simulink model "Quadcopter_close_loop"  (R2021a)
settings: Solver=ode4  StartTime=0.0  StopTime=87  FixedStep=0.001  RelTol=1e-6
values from neighbouring files (symbols this model uses):
  mean_wind = [2.72 , 1.75, -0.006]    [main_run.m]    (also in main_run_5_1.m; param_est.m = [2.72 , 1.75, .006])
  q = X(7:10)    [EKF_without_wind.m]
  r = linspace(floor(nr*0.01)/nr,1,nr)    [main_run.m]    (also in main_run_5_1.m)
  w1 = w(1)    [EKF_without_wind.m]
  x0 = [0,0,0,1,0,0,0,-P.mean_wind,0,0,0]    [main_run.m]    (also in main_run_5_1.m)
  xref = [1,1,-8,1,0,0,0,-P.mean_wind]    [main_run.m]    (also in main_run_5_1.m)
undefined symbols (not defined in the file or in its folder): HDBK, MIL, Moderate, P, u1, v1
libraries: simulink x1, aerolibwind2 x1
(part 2 of 5)

== matlab function Quadcopter_close_loop/Estimator/Estimator/IEKF_quadcopter ==
  data: sensor input; t input; y output; P parameter
function y = IEKF_quadcopter(sensor,t,P)
%% parameters 
ts = 0.01;
m = P.m;
g = P.g;
rho = P.rho;
D = P.D;
A_gr = [0;0;g];
B_i = P.B_i;

param = cell(1,6);
param{1} = A_gr;
param{2} = m;
param{3} = rho;
param{4} = D;
param{5} = ts;
param{6} = B_i;

Q_est = P.Q_est;
R_est = P.R_est;
X0_hat = P.X0_hat;
IEKF_P0 = P.IEKF_P0;
%% IEKF
persistent k P_cov X

if t >=0
    if isempty(k)
        k = 1;
        X = zeros(13,1);
        [X,P_cov] = IEKF(X0_hat,IEKF_P0,Q_est,R_est,param,sensor,k);
    end
    k = k+1;
    [X,P_cov] = IEKF(X,P_cov,Q_est,R_est,param,sensor,k);
else
    X = zeros(13,1);
end

quat = X(7:10);  
eul = quat2eul(quat')';
eul([1 3]) = eul([3 1]);
X_est = [X(1:6);eul;X(11:13)];
% Asma: Dynamics states: pos, quaternion, velocity, wind? Rearranged the dynamics so that it goes into contoller correctly 

% X_est=[X(1:3); X(7:10); X(4:6); X(11:13)];

y=X_est;
end

function [X_k1,P_k1] = IEKF(X,P,Q,R,param,sensor,iter)
% Performs one loop of the SP-EKF.
% Pre-Observer is of the form:
%   Xhat_dot = f(Xhat) + Fr*L*E*(Y - Yhat)

% Inputs:

%   X = State mean, m_k|k-1 (nx1)
%   P = State covariance, P_k|k-1(nxn)
%   f = State dynamics, xdot = f(x,param)
%   df = 
%   dh =
%   Q = Process Noise Covariance Matrix(nxn)
%   R = Measurement Noise Covariance Matrix (mxm)
%   param = Any parameters for f
%   iter = denotes the the first loop,1=yes,0=no

% Outputs:

%   X_k1 = state at next time step
%   P_k1 = state covariance at next time step

%parameter
A_gr = param{1};
m = param{2};
rho = param{3};
D = param{4};
ts = param{5};
B_i = param{6};
%sensor
% Y=[sensor{1};sensor{2};sensor{3}]; %gps+accel+B_b
% w = sensor{4};
% f_c = sensor{5};
gps = sensor(1:3);
accel = sensor(4:6);
w = sensor(7:9);
B_b = sensor(10:12);
f_c = sensor(13);

Y=[gps;accel;B_b];
U={w;f_c}; %w+f_c
%states(13*1)
x_hat=X(1:3);
vr_hat=X(4:6);
q_hat=X(7:10);
d_hat=X(11:13);

vr_hat1=vr_hat(1);vr_hat2=vr_hat(2);vr_hat3=vr_hat(3);
q_hat0=q_hat(1);q_hat1=q_hat(2);q_hat2=q_hat(3);q_hat3=q_hat(4);
%invariants
I_vr = quat_v(q_hat,vr_hat,0);
I_w = quat_v(q_hat,w,0);
b3=[0;0;1];
I_f_c = quat_v(q_hat,f_c*b3,0);
%state matrix needed for implementing the IEKF(linearized A matrix)
if norm(I_vr)==0
    mid_element=zeros(3,3);
else
%         I_D= quat_m(q_hat,D,0);
      I_D =D;
      I_D= quat_D(q_hat,D);
    mid_element =-0.5*(1/m)*rho*I_D*[norm(I_vr)+(I_vr(1)*abs(I_vr(1))*sign(I_vr(1)))/norm(I_vr)... 
                                              (I_vr(1)*abs(I_vr(2))*sign(I_vr(2)))/norm(I_vr)...
                                              (I_vr(1)*abs(I_vr(3))*sign(I_vr(3)))/norm(I_vr); ...
                                              (I_vr(2)*abs(I_vr(1))*sign(I_vr(1)))/norm(I_vr) ...
                                   norm(I_vr)+(I_vr(2)*abs(I_vr(2))*sign(I_vr(2)))/norm(I_vr) ...
                                              (I_vr(2)*abs(I_vr(3))*sign(I_vr(3)))/norm(I_vr);...
                                              (I_vr(3)*abs(I_vr(1))*sign(I_vr(1)))/norm(I_vr) ...
                                              (I_vr(3)*abs(I_vr(2))*sign(I_vr(2)))/norm(I_vr) ...
                                   norm(I_vr)+(I_vr(3)*abs(I_vr(3))*sign(I_vr(3)))/norm(I_vr);]; 
end

%dim=12x12
A_lin =@(I_vr,A_gr)[zeros(3,3)      eye(3)  -2*hat(I_vr)     eye(3);...
                    zeros(3,3) mid_element   2*hat(A_gr) zeros(3,3);...
                    zeros(3,3)  zeros(3,3)    zeros(3,3) zeros(3,3);...
                    zeros(3,3)  zeros(3,3)    zeros(3,3) zeros(3,3);]; 

%Invariant frame (13x12)
Fr =@(q_hat)[    eye(3)      zeros(3,3)      zeros(3,3) zeros(3,3);
             zeros(3,3) quat_e(q_hat,0)      zeros(3,3) zeros(3,3);
             zeros(4,3)      zeros(4,3) quat_e(q_hat,2) zeros(4,3);
             zeros(3,3)      zeros(3,3)      zeros(3,3)    eye(3);]; 
    

%T = Invariant Output Matrix, (9x9)
T =@(q_hat) [    eye(3)          zeros(3,3)    zeros(3,3);
             zeros(3,3)    quat_e(q_hat,1)     zeros(3,3);
             zeros(3,3)        zeros(3,3)  quat_e(q_hat,1)]; 
         

Ln_22 = [vr_hat2*(2*q_hat0*q_hat2 + 2*q_hat1*q_hat3) + vr_hat3*(2*q_hat0*q_hat3 - 2*q_hat1*q_hat2),     - vr_hat3*(2*q_hat2^2 + 2*q_hat3^2 - 1) - vr_hat1*(2*q_hat0*q_hat2 + 2*q_hat1*q_hat3),       vr_hat2*(2*q_hat2^2 + 2*q_hat3^2 - 1) - vr_hat1*(2*q_hat0*q_hat3 - 2*q_hat1*q_hat2);
         vr_hat3*(2*q_hat1^2 + 2*q_hat3^2 - 1) - vr_hat2*(2*q_hat0*q_hat1 - 2*q_hat2*q_hat3), vr_hat1*(2*q_hat0*q_hat1 - 2*q_hat2*q_hat3) + vr_hat3*(2*q_hat0*q_hat3 + 2*q_hat1*q_hat2),     - vr_hat1*(2*q_hat1^2 + 2*q_hat3^2 - 1) - vr_hat2*(2*q_hat0*q_hat3 + 2*q_hat1*q_hat2);
         - vr_hat2*(2*q_hat1^2 + 2*q_hat2^2 - 1) - vr_hat3*(2*q_hat0*q_hat1 + 2*q_hat2*q_hat3),       vr_hat1*(2*q_hat1^2 + 2*q_hat2^2 - 1) - vr_hat3*(2*q_hat0*q_hat2 - 2*q_hat1*q_hat3), vr_hat1*(2*q_hat0*q_hat1 + 2*q_hat2*q_hat3) + vr_hat2*(2*q_hat0*q_hat2 - 2*q_hat1*q_hat3);];
Ln_23 = [ (2*q_hat0*q_hat2 + 2*q_hat1*q_hat3)/m;
         -(2*q_hat0*q_hat1 - 2*q_hat2*q_hat3)/m;
               -(2*q_hat1^2 + 2*q_hat2^2 - 1)/m;];
Ln_32 = [      q_hat2^2 + q_hat3^2 - 1/2,   q_hat0*q_hat3 - q_hat1*q_hat2, - q_hat0*q_hat2 - q_hat1*q_hat3;
         - q_hat0*q_hat3 - q_hat1*q_hat2,       q_hat1^2 + q_hat3^2 - 1/2,   q_hat0*q_hat1 - q_hat2*q_hat3;
          q_hat0*q_hat2 - q_hat1*q_hat3, - q_hat0*q_hat1 - q_hat2*q_hat3,       q_hat1^2 + q_hat2^2 - 1/2;];
% (12x10)
Ln =[   -eye(3)      zeros(3,3)    zeros(3,1) zeros(3,3);
     zeros(3,3)          Ln_22         Ln_23  zeros(3,3);
     zeros(3,3)          Ln_32     zeros(3,1) zeros(3,3);
     zeros(3,3)      zeros(3,3)    zeros(3,1)    -eye(3);]; 
 
 if iter ==1
    W=Fr(q_hat);
    W(7,:)=[];
    P = W'*P*W;
 end
%% time update 
    %continuous
    X_minus_k1 = X; %dim(X)=13x1
    P_minus_k1 = P; %dim(P)=12x12
    N=10;
    for i=1:N
    X_minus_k1 =X_minus_k1 + (ts/N).*f(X_minus_k1,U,param);
    
    %updated states and invariants
    q_hat=X_minus_k1(7:10);
    q_hat=q_hat/norm(q_hat);    
    X_minus_k1(7:10)=q_hat; %normalization
    vr_hat=X_minus_k1(4:6);
    I_vr=quat_v(q_hat,vr_hat,0);
    
    A=A_lin(I_vr,A_gr);
    P_minus_k1 = P_minus_k1 + (ts/N).*(A*P_minus_k1 + P_minus_k1*A' + Ln*Q*Ln');
    end
    X_k1 = X_minus_k1;
    P_k1 = P_minus_k1;
% measurement update 
    H= dh(X_minus_k1,U,param); %dim(H)=9x12
    R_rot = T(q_hat)*R*T(q_hat)';
    L = P_minus_k1*H'*inv(H*P_minus_k1*H' + R_rot); %dim(L)=12x9
%     L = P_minus_k1*H'*inv(H*P_minus_k1*H' + R); %dim(L)=12x9
%     X_k1 = X_minus_k1 + Fr(q_hat)*L_*T(q_hat)*(Y-H*X_minus_k1); %dim(X_k1)=13x1
    X_k1 = X_minus_k1 + Fr(q_hat)*L*T(q_hat)*(Y-h(X_minus_k1,U,param)); %dim(X_k1)=13x1
    
    q_hat=X_k1(7:10);
    q_hat=q_hat/norm(q_hat);    
    X_k1(7:10)=q_hat;
    
    P_k1 = (eye(12)-L*H)*P_minus_k1; %dim(P_k1) = 12x12
end
 
function [X_dot] = f(X,U,param)
%states
x=X(1:3);
vr=X(4:6);
q=X(7:10);
d=X(11:13);
%inputs
w=U{1};
f_c=U{2};
%parameters
A_gr = param{1};
m = param{2};
rho = param{3};
D = param{4};
ts = param{5};
B_i= param{6};
b_3=[0;0;1];
%% system dynamics
f_vr=-(1/2)*rho*D*norm(vr)*vr;
x_dot = quat_v(q,vr,0) + d;
vr_dot = cross(vr,w) + quat_v(q,A_gr,1) - (1/m)*f_c*b_3 + (1/m)*f_vr;
q_dot = (1/2)*quat_multiply(q,[0;w]);
d_dot = [0;0;0];
%% output
X_dot = [x_dot;vr_dot;q_dot;d_dot];
end

function [Y] = h(X,U,param)
%states
x=X(1:3);
vr=X(4:6);
q=X(7:10);
d=X(11:13);
%inputs
w=U{1};
f_c=U{2};
%parameters
A_gr = param{1};
m = param{2};
rho = param{3};
D = param{4};
ts = param{5};
B_i= param{6};
b_3=[0;0;1];
%%
f_vr =-(1/2)*rho*D*norm(vr)*vr;
a = - (1/m)*f_c*b_3 + (1/m)*f_vr;
B_b = quat_v(q,B_i,1);
%% ouputs
Y = [x;a;B_b];
end

function [dhdX] = dh(X,U,param) 
%states
x_hat=X(1:3);
vr_hat=X(4:6);
q_hat=X(7:10);
d_hat=X(11:13);
% x=X(1:3);
% vr=X(4:6);
% q=X(7:10);
% d=X(11:13);
%inputs
w=U{1};
f_c=U{2};
% B_i =U{3};
%parameters
A_gr = param{1};
m = param{2};
rho = param{3};
D = param{4};
B_i= param{6};
b_3=[0;0;1];
%
% if norm(vr)==0
%     mid_element=zeros(3,3);
% else
%     mid_element = -0.5*(1/m)*rho*D*[norm(vr)+(vr(1)*abs(vr(1))*sign(vr(1)))/norm(vr) ... 
%                                               (vr(1)*abs(vr(2))*sign(vr(2)))/norm(vr) ...
%                                               (vr(1)*abs(vr(3))*sign(vr(3)))/norm(vr);...
%                                               (vr(2)*abs(vr(1))*sign(vr(1)))/norm(vr) ...
%                                    norm(vr)+(vr(2)*abs(vr(2))*sign(vr(2)))/norm(vr) ...
%                                               (vr(2)*abs(vr(3))*sign(vr(3)))/norm(vr);...
%                                               (vr(3)*abs(vr(1))*sign(vr(1)))/norm(vr) ...
%                                               (vr(3)*abs(vr(2))*sign(vr(2)))/norm(vr) ...
%                                    norm(vr)+(vr(3)*abs(vr(3))*sign(vr(3)))/norm(vr);]; 
% end
% %dim=9x12           
% dhdX = [    eye(3)  zeros(3,3)  zeros(3,3) zeros(3,3);
%         zeros(3,3) mid_element  zeros(3,3) zeros(3,3);
%         zeros(3,3) zeros(3,3)  2*hat(B_i) zeros(3,3);];

%invariants
I_vr = quat_v(q_hat,vr_hat,0);
if norm(I_vr)==0
    mid_element=zeros(3,3);
else
%         I_D= quat_m(q_hat,D,0);
%       I_D=D;
      I_D= quat_D(q_hat,D);
    mid_element =-0.5*(1/m)*rho*I_D*[norm(I_vr)+(I_vr(1)*abs(I_vr(1))*sign(I_vr(1)))/norm(I_vr)... 
                                              (I_vr(1)*abs(I_vr(2))*sign(I_vr(2)))/norm(I_vr)...
                                              (I_vr(1)*abs(I_vr(3))*sign(I_vr(3)))/norm(I_vr); ...
                                              (I_vr(2)*abs(I_vr(1))*sign(I_vr(1)))/norm(I_vr) ...
                                   norm(I_vr)+(I_vr(2)*abs(I_vr(2))*sign(I_vr(2)))/norm(I_vr) ...
                                              (I_vr(2)*abs(I_vr(3))*sign(I_vr(3)))/norm(I_vr);...
                                              (I_vr(3)*abs(I_vr(1))*sign(I_vr(1)))/norm(I_vr) ...
                                              (I_vr(3)*abs(I_vr(2))*sign(I_vr(2)))/norm(I_vr) ...
                                   norm(I_vr)+(I_vr(3)*abs(I_vr(3))*sign(I_vr(3)))/norm(I_vr);]; 
end
%dim=9x12           
dhdX = [   eye(3)  zeros(3,3)  zeros(3,3) zeros(3,3);
        zeros(3,3) mid_element  zeros(3,3) zeros(3,3);
        zeros(3,3) zeros(3,3)  2*hat(B_i) zeros(3,3);];
end

%% quaternion library
function new_D=quat_D(q,D)
      q0=q(1);
      qv=q(2:4);
      R=eye(3)+2*q0*hat(qv)+2*hat(qv)*hat(qv);
      new_D=R*D*R';
end

function vec=quat_v(q,v,type)
    if type == 0 %q*v*q^-1
      q0=q(1);
      qv=q(2:4);
      R=eye(3)+2*q0*hat(qv)+2*hat(qv)*hat(qv);
      vec=R*v;
    elseif type == 1 %q^-1*v*q
      q0=q(1);
      qv=q(2:4);
      R=eye(3)+2*q0*hat(qv)+2*hat(qv)*hat(qv);
      vec=inv(R)*v;
    end
end

== matlab function Quadcopter_close_loop/Estimator/sensors/sensors ==
  settings: updateMethod=DISCRETE
  data: x input; x_dot input; P parameter; Accel_Gyro output; B_b output
function [Accel_Gyro,B_b] = fcn(x,x_dot,P)
%#codegen

% veocity 8-10
Pn_ddot = x_dot(8);
Pe_ddot = x_dot(9);
Pd_ddot = x_dot(10);

% phi = x(7);
% theta = x(8);
% psi = x(9);

% Hao please check if this is right
quat_angle = x(4:7);
eul = quat2eul(quat_angle')';
eul([1 3]) = eul([3 1]); %Hao
phi = eul(1);
theta = eul(2);
psi = eul(3);

p = x(11);
q = x(12);
r = x(13);

g = P.g ;

bias_gyro_x=P.bias_gyro_x;
bias_gyro_y=P.bias_gyro_y;
bias_gyro_z=P.bias_gyro_z;
sigma_gyro =P.sigma_gyro;

bias_accel_x = P.bias_accel_x;
bias_accel_y = P.bias_accel_y;
bias_accel_z = P.bias_accel_z;
sigma_accel = P.sigma_accel;

bias_B_x = P.bias_B_x;
bias_B_y = P.bias_B_y;
bias_B_z = P.bias_B_z;
sigma_B = P.sigma_B;
% simulate rate gyros (units are rad/sec)
y_gyro_x = p + bias_gyro_x + sigma_gyro*randn;
y_gyro_y = q + bias_gyro_y + sigma_gyro*randn;
y_gyro_z = r + bias_gyro_z + sigma_gyro*randn;

% simulate accelerometers (units of g)
Pd_ddot = Pd_ddot- g;
P_ddot=[Pn_ddot;Pe_ddot;Pd_ddot];
%rotation matrix which can rotate the vector from inertial frame to body
%frame
Rbi=[                          cos(theta)*cos(psi)                            cos(theta)*sin(psi)         -sin(theta);
    sin(phi)*sin(theta)*cos(psi)-cos(phi)*sin(psi) sin(phi)*sin(theta)*sin(psi)+cos(phi)*cos(psi) sin(phi)*cos(theta);
    cos(phi)*sin(theta)*cos(psi)+sin(phi)*sin(psi) cos(phi)*sin(theta)*sin(psi)-sin(phi)*cos(psi) cos(phi)*cos(theta)];

a=Rbi*P_ddot;
ax=a(1);ay=a(2);az=a(3);
y_accel_x = ax + bias_accel_x + sigma_accel*randn;
y_accel_y = ay + bias_accel_y + sigma_accel*randn;
y_accel_z = az + bias_accel_z + sigma_accel*randn;

Accel_Gyro =[y_accel_x;
             y_accel_y;
             y_accel_z;
             y_gyro_x;
             y_gyro_y;
             y_gyro_z;];

%simulate the Magnetometer sensor
% B_i=[1/sqrt(2);0;1/sqrt(2)];
B_i = P.B_i;

B_b=Rbi*B_i;
B_b(1) = B_b(1) + bias_B_x + sigma_B*randn;
B_b(2) = B_b(2) + bias_B_y + sigma_B*randn;
B_b(3) = B_b(3) + bias_B_z + sigma_B*randn;
end
